simulink model "Fig56"  (R2014b)
settings: Solver=ode3  StartTime=0.0  StopTime=10.001  FixedStep=2e-6  RelTol=1e-5
libraries: commsink2 x3, commfilt2 x3, commrandsrc2 x3, commanapbnd3 x2, commchan3 x1
settings Model: Creator=Dennis Silage  LastModifiedBy=Silage
settings DataIOCC: SignalLoggingSaveFormat=ModelDataLogs
settings OptimizationCC: ExpressionDepthLimit=2147483647  InitFltsAndDblsToZero=on
settings DebuggingCC: UnderspecifiedInitializationDetection=Classic  MergeDetectMultiDrivingBlocksExec=none  SolverPrmCheckMsg=none  FcnCallInpInsideContextMsg=UseLocalSettings  StateNameClashWarn=warning
settings GRTTargetCC: CombineOutputUpdateFcns=off  GRTInterface=on

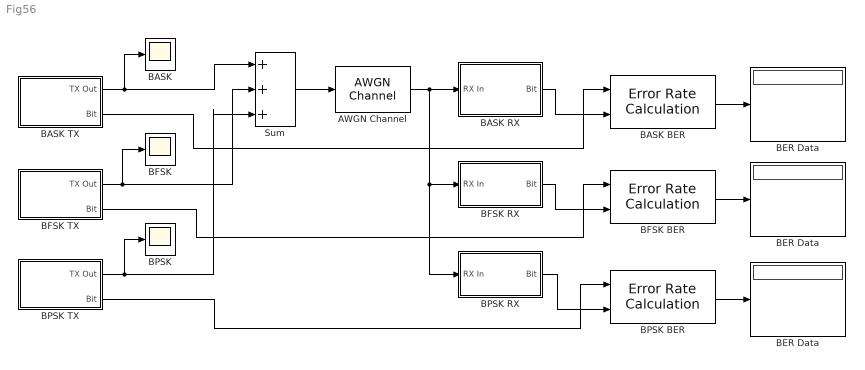
== system Fig56 ==
  AWGN Channel : commchan3/AWGN Channel  InputProcessing=Inherited (this choice will be removed - see release notes)  seed=randseed  noiseMode="Signal to noise ratio  (Eb/No)"  EbNodB=80  EsNodB=10  SNRdB=12  bitsPerSym=1  Ps=12.5  Tsym=1e-3  variance=0
  BASK : Scope
      settings: YMin=-6  YMax=6
  BASK BER : commsink2/Error Rate Calculation  N=2  st_delay=0  cp_mode=Entire frame  subframe=[]  PMode=Port  WsName=ErrorVec  RsMode2=off  stop=off  numErr=100  maxBits=1e6
  BASK RX : Subsystem
  BASK TX : Subsystem
  BER Data : Display
  "BER Data " : Display
  "BER Data  " : Display
  BFSK : Scope
      settings: TimeRange=0.005  YMin=-6  YMax=6
  BFSK BER : commsink2/Error Rate Calculation  N=2  st_delay=0  cp_mode=Entire frame  subframe=[]  PMode=Port  WsName=ErrorVec  RsMode2=off  stop=off  numErr=100  maxBits=1e6
  BFSK RX : Subsystem
  BFSK TX : Subsystem
  BPSK : Scope
      settings: YMin=-6  YMax=6  SaveName=ScopeData2
  BPSK BER : commsink2/Error Rate Calculation  N=2  st_delay=0  cp_mode=Entire frame  subframe=[]  PMode=Port  WsName=ErrorVec  RsMode2=off  stop=off  numErr=100  maxBits=1e6
  BPSK RX : Subsystem
  BPSK TX : Subsystem
  Sum : Sum  Inputs=|+|+|+|
  wires:
  BASK BER/1 -> BER Data/1
  BASK TX/1(TX Out) -> Sum/1, BASK/1
  BASK TX/2(Bit) -> BASK BER/1
  AWGN Channel/1 -> BPSK RX/1(RX In), BFSK RX/1(RX In), BASK RX/1(RX In)
  BASK RX/1(Bit) -> BASK BER/2
  BFSK TX/1(TX Out) -> BFSK/1, Sum/2
  BFSK TX/2(Bit) -> BFSK BER/1
  BFSK RX/1(Bit) -> BFSK BER/2
  BFSK BER/1 -> "BER Data "/1
  BPSK TX/1(TX Out) -> Sum/3, BPSK/1
  BPSK TX/2("Bit ") -> BPSK BER/1
  BPSK RX/1(Bit) -> BPSK BER/2
  BPSK BER/1 -> "BER Data  "/1
  Sum/1 -> AWGN Channel/1

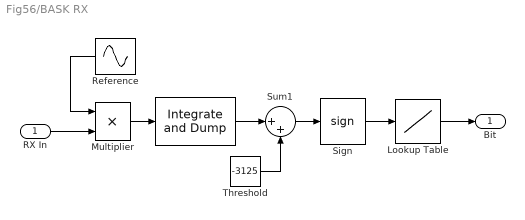
== system Fig56/BASK RX ==
  RX In : Inport
  " " : commfilt2/Integrate and Dump  obssamples=500  offsetsamples=0  nodump=off  roundingMode=Floor  overflowMode=off
  Lookup Table : Lookup_n-D  NumberOfTableDimensions=1  BreakpointsForDimension1=[-1, 0, 1]  BreakpointsForDimension3=[5, 7]  Table=[0, 0, 1]  InternalRulePriority=Speed  RndMeth=Simplest  InputSameDT=on
  Multiplier : Product  RndMeth=Zero
  Reference : Sin  Amplitude=5  Frequency=31000*pi  Samples=200  SampleTime=2e-6
  Sign : Signum
  Sum1 : Sum  Inputs=|++
  Threshold : Constant  Value=-3125
  Bit : Outport
  wires:
  Sign/1 -> Lookup Table/1
  Multiplier/1 -> " "/1
  RX In/1 -> Multiplier/2
  Threshold/1 -> Sum1/2
  Sum1/1 -> Sign/1
  " "/1 -> Sum1/1
  Reference/1 -> Multiplier/1
  Lookup Table/1 -> Bit/1

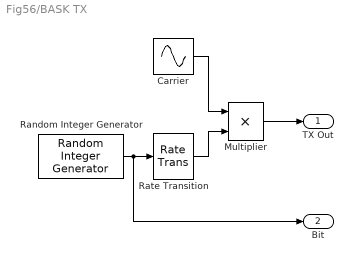
== system Fig56/BASK TX ==
  Carrier : Sin  Amplitude=5  Frequency=31000*pi  SampleTime=2e-6
  "Multiplier " : Product  RndMeth=Zero
  Random Integer Generator : commrandsrc2/Random Integer Generator  mul=2  seed=randseed  Ts=1e-3  frameBased=off  sampPerFrame=50  orient=on  outDataType=double
  Rate Transition : RateTransition  OutPortSampleTime=2e-6
  TX Out : Outport
  Bit : Outport  Port=2
  wires:
  Random Integer Generator/1 -> Bit/1, Rate Transition/1
  "Multiplier "/1 -> TX Out/1
  Carrier/1 -> "Multiplier "/1
  Rate Transition/1 -> "Multiplier "/2

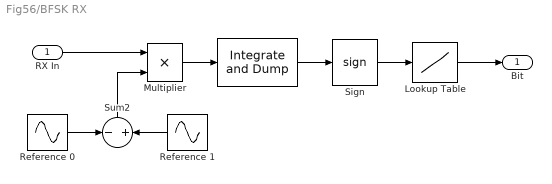
== system Fig56/BFSK RX ==
  RX In : Inport
  " " : commfilt2/Integrate and Dump  obssamples=500  offsetsamples=0  nodump=off  roundingMode=Floor  overflowMode=off
  Lookup Table : Lookup_n-D  NumberOfTableDimensions=1  BreakpointsForDimension1=[-1, 0, 1]  BreakpointsForDimension3=[5, 7]  Table=[0, 0, 1]  InternalRulePriority=Speed  RndMeth=Simplest  InputSameDT=on
  Multiplier : Product  RndMeth=Zero
  Reference 0 : Sin  Amplitude=5  Frequency=39000*pi  Phase=pi/2  Samples=200  SampleTime=2e-6
  Reference 1 : Sin  Amplitude=5  Frequency=41000*pi  Phase=pi/2  Samples=200  SampleTime=2e-6
  Sign : Signum
  Sum2 : Sum  Inputs=-+
  Bit : Outport
  wires:
  RX In/1 -> Multiplier/1
  Multiplier/1 -> " "/1
  Sign/1 -> Lookup Table/1
  Reference 1/1 -> Sum2/2
  Reference 0/1 -> Sum2/1
  " "/1 -> Sign/1
  Sum2/1 -> Multiplier/2
  Lookup Table/1 -> Bit/1

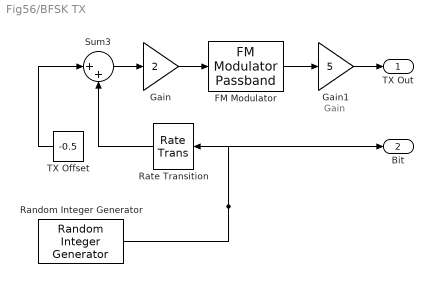
== system Fig56/BFSK TX ==
  note: Gain
  FM Modulator : commanapbnd3/FM Modulator Passband  Fc=20000  Ph=0  Kc=500
  Gain : Gain  Gain=2
  Gain1 : Gain  Gain=5
  Random Integer Generator : commrandsrc2/Random Integer Generator  mul=2  seed=46  Ts=1e-3  frameBased=off  sampPerFrame=50  orient=on  outDataType=double
  Rate Transition : RateTransition  OutPortSampleTime=2e-6
  Sum3 : Sum  Inputs=|++
  TX Offset : Constant  Value=-0.5
  TX Out : Outport
  Bit : Outport  Port=2
  wires:
  Sum3/1 -> Gain/1
  TX Offset/1 -> Sum3/1
  Random Integer Generator/1 -> Bit/1, Rate Transition/1
  Rate Transition/1 -> Sum3/2
  Gain/1 -> FM Modulator/1
  FM Modulator/1 -> Gain1/1
  Gain1/1 -> TX Out/1

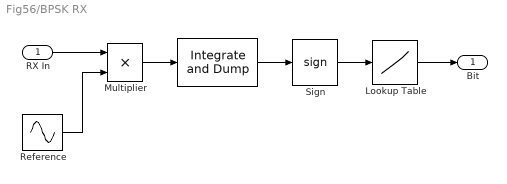
== system Fig56/BPSK RX ==
  RX In : Inport
  " " : commfilt2/Integrate and Dump  obssamples=500  offsetsamples=0  nodump=off  roundingMode=Floor  overflowMode=off
  " Lookup Table" : Lookup_n-D  NumberOfTableDimensions=1  BreakpointsForDimension1=[-1, 0, 1]  BreakpointsForDimension3=[5, 7]  Table=[0, 0, 1]  InternalRulePriority=Speed  RndMeth=Simplest  InputSameDT=on
  Multiplier : Product  RndMeth=Zero
  Reference : Sin  Amplitude=5  Frequency=49000*pi  Phase=pi/2  Samples=200  SampleTime=2e-6
  Sign : Signum
  Bit : Outport
  wires:
  Sign/1 -> " Lookup Table"/1
  Multiplier/1 -> " "/1
  " Lookup Table"/1 -> Bit/1
  " "/1 -> Sign/1
  Reference/1 -> Multiplier/2
  RX In/1 -> Multiplier/1

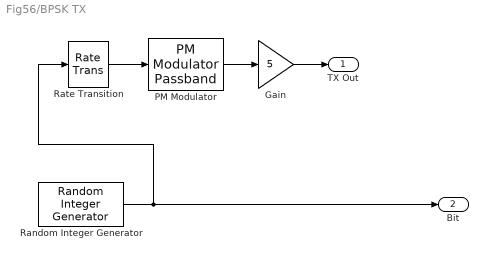
== system Fig56/BPSK TX ==
  Gain : Gain  Gain=5
  PM Modulator : commanapbnd3/PM Modulator Passband  Fc=24500  Ph=pi  Kc=pi
  Random Integer Generator : commrandsrc2/Random Integer Generator  mul=2  seed=randseed  Ts=1e-3  frameBased=off  sampPerFrame=50  orient=on  outDataType=double
  Rate Transition : RateTransition  OutPortSampleTime=2e-6
  TX Out : Outport
  "Bit " : Outport  Port=2
  wires:
  PM Modulator/1 -> Gain/1
  Rate Transition/1 -> PM Modulator/1
  Gain/1 -> TX Out/1
  Random Integer Generator/1 -> "Bit "/1, Rate Transition/1
